simulink model "wk4sim_nonlinear"  (R2021b)
settings: Solver=VariableStepAuto  StartTime=0.0  StopTime=10.0  RelTol=1e-3
undefined symbols (not defined in the file): g, L, m, Mc, x0
settings Model: Creator=Cyril  LastModifiedBy=Cyril

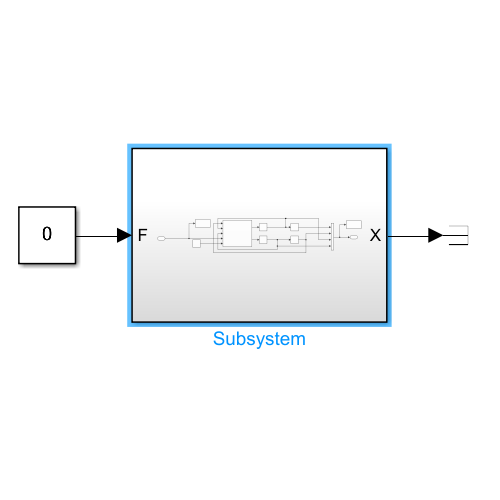
[thumbnail: Simulink's stored preview of the top-level diagram]
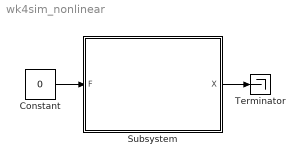
== system wk4sim_nonlinear ==
  Constant : Constant  Value=0
  Subsystem : Subsystem
  Terminator : Terminator
  wires:
  Subsystem/1(X) -> Terminator/1
  Constant/1 -> Subsystem/1(F)

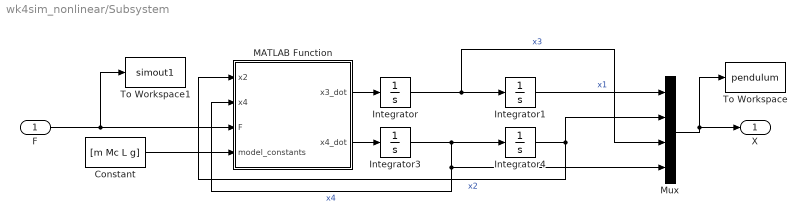
== system wk4sim_nonlinear/Subsystem ==
  F : Inport
  Constant : Constant  Value=[m Mc L g]
  Integrator : Integrator  InitialCondition=x0(3)
  Integrator1 : Integrator  InitialCondition=x0(1)
  Integrator3 : Integrator  InitialCondition=x0(4)
  Integrator4 : Integrator  InitialCondition=x0(2)
  MATLAB Function : MATLAB Function  TreatAsAtomicUnit=on
  Mux : Mux
  To Workspace : ToWorkspace  VariableName=pendulum  SampleTime=-1
  To Workspace1 : ToWorkspace  VariableName=simout1  SampleTime=-1
  X : Outport
  wires:
  MATLAB Function/2(x4_dot) -> Integrator3/1
  Constant/1 -> MATLAB Function/4(model_constants)
  Integrator1/1 -> Mux/1  "x1"
  Integrator4/1 -> Mux/2, MATLAB Function/1(x2)  "x2"
  MATLAB Function/1(x3_dot) -> Integrator/1
  Mux/1 -> To Workspace/1, X/1
  Integrator/1 -> Integrator1/1, Mux/3  "x3"
  Integrator3/1 -> Integrator4/1, MATLAB Function/2(x4), Mux/4  "x4"
  F/1 -> MATLAB Function/3(F), To Workspace1/1

== matlab function wk4sim_nonlinear/Subsystem/MATLAB Function ==
  data: x2 input; x3_dot output; x4 input; F input; model_constants input; x4_dot output
function [x3_dot, x4_dot]= nonlineqn(x2, x4, F, model_constants)

m = model_constants(1);
Mc = model_constants(2);
L = model_constants(3);
g = model_constants(4);

x3_dot = (((x4)^2 * L * m * sin(x2)) - (g * m * sin(x2) * cos(2)) + F) / (Mc + m - (m * cos(x2)^2));
x4_dot = ((-1 * L * m * sin(x2) * cos(x2) * (x4)^2) + (g * (Mc + m) * sin(x2)) - (cos(x2) * F)) / (L * (Mc + m - (m * cos(x2)^2)));
